simulink library "INT_PthSet_OvrRunCoord"  (R2016b)
settings: Solver=VariableStepAuto  StartTime=0.0  StopTime=10.0  RelTol=1e-3
settings Model: Creator=Administrator  LastModifiedBy=Administrator

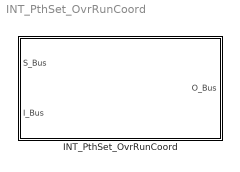
== system INT_PthSet_OvrRunCoord ==
  INT_PthSet_OvrRunCoord : Subsystem

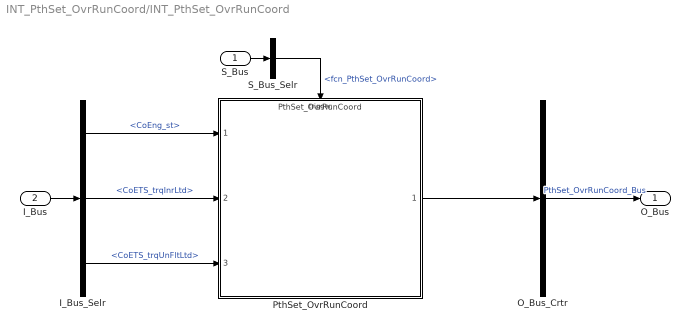
== system INT_PthSet_OvrRunCoord/INT_PthSet_OvrRunCoord ==
  S_Bus : Inport
  I_Bus : Inport  Port=2
  I_Bus_Selr : BusSelector  OutputSignals=CoEng_st,CoETS_trqInrLtd,CoETS_trqUnFltLtd
  O_Bus_Crtr : BusCreator  Inputs=1
  PthSet_OvrRunCoord : ModelReference  ModelNameDialog=PthSet_OvrRunCoord  SimulationMode=Normal  ModelReferenceVersion=1.2  TriggerPortName=function  TriggerPortTriggerType=function-call  TriggerPortStatesWhenEnabling=held
  S_Bus_Selr : BusSelector  OutputSignals=fcn_PthSet_OvrRunCoord
  O_Bus : Outport
  wires:
  S_Bus_Selr/1 -> PthSet_OvrRunCoord/Trigger  "<fcn_PthSet_OvrRunCoord>"
  S_Bus/1 -> S_Bus_Selr/1
  I_Bus/1 -> I_Bus_Selr/1
  I_Bus_Selr/1 -> PthSet_OvrRunCoord/1  "<CoEng_st>"
  I_Bus_Selr/2 -> PthSet_OvrRunCoord/2  "<CoETS_trqInrLtd>"
  I_Bus_Selr/3 -> PthSet_OvrRunCoord/3  "<CoETS_trqUnFltLtd>"
  O_Bus_Crtr/1 -> O_Bus/1  "PthSet_OvrRunCoord_Bus"
  PthSet_OvrRunCoord/1 -> O_Bus_Crtr/1
